simulink model "GFLGFM"  (R2022a)
settings: Solver=FixedStepAuto  StartTime=0.0  StopTime=3  FixedStep=Ts  RelTol=1e-3
values from neighbouring files (symbols this model uses):
  Cf1 = 0.002    [GFLGFM_Para.m]
  Cf2 = 0.2    [GFLGFM_Para.m]
  dt_jump = 2    [GFLGFM_Para.m]    (also in GFLGSP_Para.m)
  dt_sag = 0.01    [GFLGFM_Para.m]    (also in GFLGSP_Para.m)
  ki_pll1 = 0    [GFLGFM_Para.m]    (also in GFLGSP_Para.m)
  kp_pll1 = w_pll1    [GFLGFM_Para.m]    (also in GFLGSP_Para.m)
  L1 = X1    [GFLGFM_Para.m]    (also in GFLGSP_Para.m)
  L2 = X2    [GFLGFM_Para.m]    (also in GFLGSP_Para.m)
  Lc1 = 1e-9    (= 1e-09)    [GFLGFM_Para.m]
  Lc2 = 1e-9    (= 1e-09)    [GFLGFM_Para.m]
  Lf1 = 0.1    [GFLGFM_Para.m]
  Lf2 = 0.1    [GFLGFM_Para.m]
  Lg = Xg    [GFLGFM_Para.m]    (also in GFLGSP_Para.m)
  M = Kgfm/Wbase    [GFLGFM_Para.m]
  phase_jump = -1.2    [GFLGFM_Para.m]    (also in GFLGSP_Para.m)
  Pm = Pref    [GFLGFM_Para.m]
  position = position    [GFLGSP_Para.m]
  R1 = R1    [GFLGFM_Para.m]    (also in GFLGSP_Para.m)
  R2 = R2    [GFLGFM_Para.m]    (also in GFLGSP_Para.m)
  Rg = Rg    [GFLGFM_Para.m]    (also in GFLGSP_Para.m)
  Sbase = 1    [GFLGFM_Para.m]    (also in GFLGSP_Para.m)
  Scale_ki_v = 60    [GFLGFM_Para.m]
  t0 = 2    [GFLGFM_Para.m]    (also in GFLGSP_Para.m = 2.5)
  t0_jump = 10    [GFLGFM_Para.m]    (also in GFLGSP_Para.m)
  t0_sag = 10    [GFLGFM_Para.m]    (also in GFLGSP_Para.m)
  tc1 = t_c    [GFLGFM_Para.m]    (also in GFLGSP_Para.m = t_c-0.01)
  tc2 = t_c2    [GFLGFM_Para.m]    (also in GFLGSP_Para.m = t_c)
  Ts = 1/Fs    (= 1e-05)    [GFLGFM_Para.m]    (also in GFLGSP_Para.m)
  v_sag = 0.1    [GFLGFM_Para.m]    (also in GFLGSP_Para.m)
  Vbase = 1    [GFLGFM_Para.m]    (also in GFLGSP_Para.m)
  w_droop = 15*2*pi    (= 94.2477796077)    [GFLGFM_Para.m]
  w_i_GFL1 = 2500 *2*pi    (= 15707.9632679)    [GFLGFM_Para.m]    (also in GFLGSP_Para.m = 6283.18530718)
  w_i_GFM = 2500*2*pi    (= 15707.9632679)    [GFLGFM_Para.m]
  w_pll1 = k1p    [GFLGFM_Para.m]    (also in GFLGSP_Para.m)
  w_tau1 = 1e3*2*pi    (= 6283.18530718)    [GFLGFM_Para.m]    (also in GFLGSP_Para.m)
  w_v_GFM = 200 *2*pi    (= 1256.63706144)    [GFLGFM_Para.m]
  Wbase = 2*pi*50    (= 314.159265359)    [GFLGFM_Para.m]    (also in GFLGSP_Para.m)
  Zbase = Vbase/Ibase    (= 1)    [GFLGFM_Para.m]    (also in GFLGSP_Para.m)
undefined symbols (not defined in the file or in its folder): DiscIntNeverNeededParam, I1d, I1q, initial
libraries: spsVoltageMeasurementLib x96, spsCurrentMeasurementLib x78, SimplexPS x36, spsThreePhaseSeriesRLCBranchLib x34, spsControlledVoltageSourceLib x30, SimplexPS_2015a x12, spsGroundLib x7, spsSeriesRLCBranchLib x6, spsThreePhaseBreakerLib x4, spsMultimeterLib x2, spsThreePhaseFaultLib x2, spspowerguiLib x1
(part 1 of 6)
settings Model: Creator=admin_user  LastModifiedBy=yz7521
settings SolverCC: AlgebraicLoopSolver=TrustRegion
settings DataIOCC: ReturnWorkspaceOutputs=off
settings DebuggingCC: UnconnectedInputMsg=warning  UnconnectedOutputMsg=warning  UnconnectedLineMsg=warning  SFMachineParentedDataDiag=warning
settings RTWCC: DLArmComputeVersion=19.05

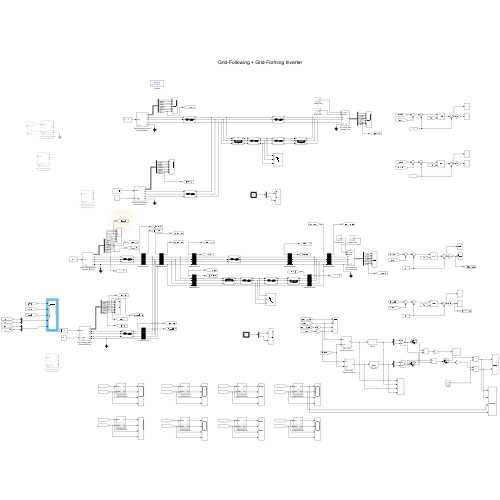
[thumbnail: Simulink's stored preview of the top-level diagram]
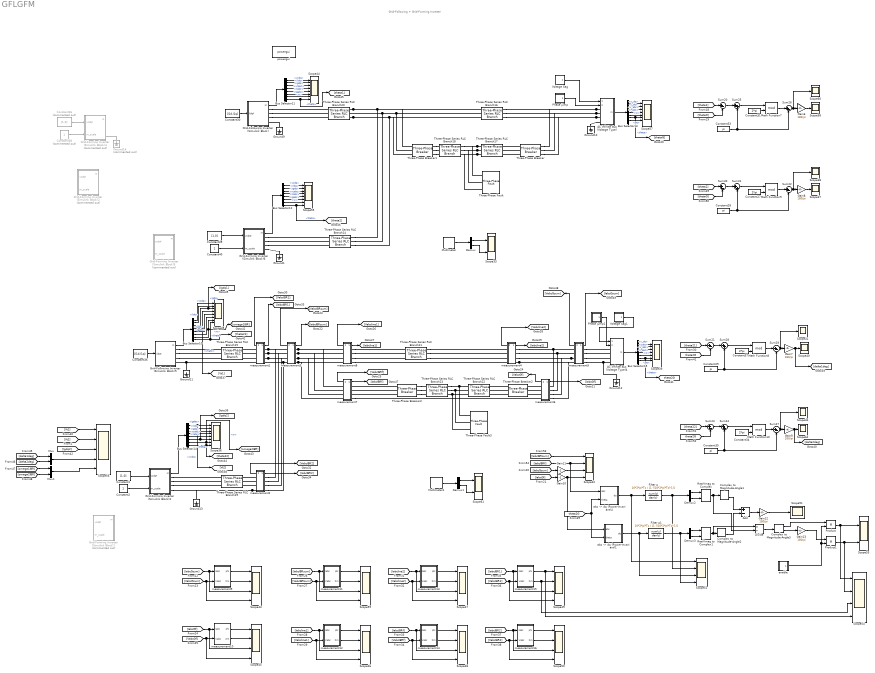
== system GFLGFM ==
  note: Grid-Following + Grid-Forming Inverter
  AC Infinite Bus (Voltage Type) : Subsystem  AncestorBlock=|  mask{Ts=Ts, Sbase=Sbase, Vbase=Vbase, Wbase=Wbase, theta0=0, w=Wbase, R=1e-30}
      | SimplusGT/AC Infinite Bus
      | (Voltage Type)
      mask prompts: Ts "Ts (s), samping period"; Sbase "Sbase (VA), power base"; Vbase "Vbase (V), voltage base"; Wbase "Wbase (rad/s), frequency base"; theta0 "theta0 (rad), initial angle"; w "w (rad/s), frequency"; R "R (Ohm), resistance"
  AC Infinite Bus (Voltage Type)4 : Subsystem  AncestorBlock=|  mask{Ts=Ts, Sbase=Sbase, Vbase=Vbase, Wbase=Wbase, theta0=0, w=Wbase, R=1e-30}
      | SimplusGT/AC Infinite Bus
      | (Voltage Type)
      mask prompts: Ts "Ts (s), samping period"; Sbase "Sbase (VA), power base"; Vbase "Vbase (V), voltage base"; Wbase "Wbase (rad/s), frequency base"; theta0 "theta0 (rad), initial angle"; w "w (rad/s), frequency"; R "R (Ohm), resistance"
  Add : Sum  Inputs=+-
  Bus Selector{10..12,14} (4 alike) : BusSelector  OutputSignals=vcdq,ildq,igdq,vcabc,ilabc,igabc,w,theta
  Bus Selector13 : BusSelector  OutputSignals=v_dq,i_dq,v_abc,i_abc,w,theta,pq
  Bus Selector15 : BusSelector  OutputSignals=v_dq,i_dq,v_abc,i_abc,w,theta,pq
  Complex to Magnitude-Angle1 : ComplexToMagnitudeAngle
  Complex to Magnitude-Angle2 : ComplexToMagnitudeAngle
  Complex to Magnitude-Angle3 : ComplexToMagnitudeAngle
  Constant1 : Constant  Value=[1,0]
  Constant2 : Constant
  Constant26 : Constant  Commented=on  Value=[1,0]
  Constant{27,31,34,37} (4 alike) : Constant  Value=2*pi
  Constant{28..29,33,35} (4 alike) : Constant  Value=pi
  Constant30 : Constant  Value=[I1d,I1q]
  Constant36 : Constant  Value=[I1d,I1q]
  Constant38 : Constant  Commented=on
  Constant39 : Constant  Value=[1,0]
  Constant40 : Constant
  Demux : Demux  Outputs=[3 3]
  Demux1 : Demux  Outputs=[3 3]
  Demux2 : Demux  Outputs=2
  Demux3 : Demux  Outputs=2
  Divide : Product  Inputs=*/
  Filter p : DiscreteTransferFcn  Numerator=10*2*pi*Ts  Denominator=[1 ((10*2*pi*Ts)-1)]  SampleTime=Ts
  Filter p1 : DiscreteTransferFcn  Numerator=10*2*pi*Ts  Denominator=[1 ((10*2*pi*Ts)-1)]  SampleTime=Ts
  Gain10 : Gain  Gain=-1
  Gain11 : Gain  Gain=-1
  Gain{6..9,12..13} (6 alike) : Gain  Gain=180/pi
  Grid-Following Inverter (Simulink Block) : Subsystem  AncestorBlock=|  mask{Ts=Ts, Sbase=Sbase, Vbase=Vbase, Wbase=Wbase, w_i=w_i_GFL1, w_pll=w_pll1, w_tau=w_tau1, Lf=Lf1, Cf=Cf1, Lc=Lc1}
      | SimplusGT/Grid-Following Inverter
      | (Simulink Block)
      mask prompts: Ts "Ts (s), sampling period"; Sbase "Sbase (VA), base power"; Vbase "Vbase (V), base voltage"; Wbase "Wbase (rad/s), base frequency"; w_i "w_i (rad/s), current-loop bandwidth"; w_pll "w_pll (rad/s), PLL bandwidth"; w_tau "w_tau (rad/s), PLL filter bandwidth"; Lf "Lf (pu), LCL filter"; Cf "Cf (pu), LCL filter"; Lc "Lc (pu), LCL filter"
  Grid-Following Inverter (Simulink Block)5 : Subsystem  AncestorBlock=|  mask{Ts=Ts, Sbase=Sbase, Vbase=Vbase, Wbase=Wbase, w_i=w_i_GFL1, w_pll=w_pll1, w_tau=w_tau1, Lf=Lf1, Cf=Cf1, Lc=Lc1}
      | SimplusGT/Grid-Following Inverter
      | (Simulink Block)
      mask prompts: Ts "Ts (s), sampling period"; Sbase "Sbase (VA), base power"; Vbase "Vbase (V), base voltage"; Wbase "Wbase (rad/s), base frequency"; w_i "w_i (rad/s), current-loop bandwidth"; w_pll "w_pll (rad/s), PLL bandwidth"; w_tau "w_tau (rad/s), PLL filter bandwidth"; Lf "Lf (pu), LCL filter"; Cf "Cf (pu), LCL filter"; Lc "Lc (pu), LCL filter"
  Grid-Forming Inverter (Simulink Block)1 : Subsystem  Commented=on  AncestorBlock=|  mask{Ts=Ts, Sbase=Sbase, Vbase=Vbase, Wbase=Wbase, w_i=w_i_GFM, w_v=w_v_GFM, w_droop=w_droop*1, m=M*1, Lf=Lf2, Cf=Cf2, Lc=Lc2, Scale_ki_v=Scale_ki_v}
      | SimplexPS/Grid-Forming Inverter
      | (Simulink Block)
      mask prompts: Ts "Ts (s), sampling period"; Sbase "Sbase (VA), base power"; Vbase "Vbase (V), base voltage"; Wbase "Wbase (rad/s), base frequency"; w_i "w_i (rad/s), current-loop bandwidth"; w_v "w_v (rad/s), voltage-loop bandwidth"; w_droop "w_droop (rad/s), droop bandwidth"; m "m (pu), frequency droop gain"; Lf "Lf (pu), LCL filter"; Cf "Cf (pu), LCL filter"; Lc "Lc (pu), LCL filter"
  Grid-Forming Inverter (Simulink Block)2 : Subsystem  Commented=on  AncestorBlock=|  mask{Ts=Ts, Sbase=Sbase, Vbase=Vbase, Wbase=Wbase, w_i=w_i_GFM, w_v=w_v_GFM, w_droop=w_droop*1, m=M*1, Lf=Lf2, Cf=Cf2, Lc=Lc2, Scale_ki_v=Scale_ki_v}
      | SimplexPS/Grid-Forming Inverter
      | (Simulink Block)
      mask prompts: Ts "Ts (s), sampling period"; Sbase "Sbase (VA), base power"; Vbase "Vbase (V), base voltage"; Wbase "Wbase (rad/s), base frequency"; w_i "w_i (rad/s), current-loop bandwidth"; w_v "w_v (rad/s), voltage-loop bandwidth"; w_droop "w_droop (rad/s), droop bandwidth"; m "m (pu), frequency droop gain"; Lf "Lf (pu), LCL filter"; Cf "Cf (pu), LCL filter"; Lc "Lc (pu), LCL filter"
  Grid-Forming Inverter (Simulink Block)3 : Subsystem  AncestorBlock=|  mask{Ts=Ts, Sbase=Sbase, Vbase=Vbase, Wbase=Wbase, w_i=w_i_GFM, w_v=w_v_GFM, w_droop=w_droop*1, m=M*1, Lf=Lf2, Cf=Cf2, Lc=Lc2, Scale_ki_v=Scale_ki_v}
      | SimplexPS/Grid-Forming Inverter
      | (Simulink Block)
      mask prompts: Ts "Ts (s), sampling period"; Sbase "Sbase (VA), base power"; Vbase "Vbase (V), base voltage"; Wbase "Wbase (rad/s), base frequency"; w_i "w_i (rad/s), current-loop bandwidth"; w_v "w_v (rad/s), voltage-loop bandwidth"; w_droop "w_droop (rad/s), droop bandwidth"; m "m (pu), frequency droop gain"; Lf "Lf (pu), LCL filter"; Cf "Cf (pu), LCL filter"; Lc "Lc (pu), LCL filter"
  Grid-Forming Inverter (Simulink Block)4 : Subsystem  Commented=on  AncestorBlock=|  mask{Ts=Ts, Sbase=Sbase, Vbase=Vbase, Wbase=Wbase, w_i=w_i_GFM, w_v=w_v_GFM, w_droop=w_droop*1, m=M*1, Lf=Lf2, Cf=Cf2, Lc=Lc2, Scale_ki_v=Scale_ki_v}
      | SimplexPS/Grid-Forming Inverter
      | (Simulink Block)
      mask prompts: Ts "Ts (s), sampling period"; Sbase "Sbase (VA), base power"; Vbase "Vbase (V), base voltage"; Wbase "Wbase (rad/s), base frequency"; w_i "w_i (rad/s), current-loop bandwidth"; w_v "w_v (rad/s), voltage-loop bandwidth"; w_droop "w_droop (rad/s), droop bandwidth"; m "m (pu), frequency droop gain"; Lf "Lf (pu), LCL filter"; Cf "Cf (pu), LCL filter"; Lc "Lc (pu), LCL filter"
  Grid-Forming Inverter (Simulink Block)5 : Subsystem  Commented=on  AncestorBlock=|  mask{Ts=Ts, Sbase=Sbase, Vbase=Vbase, Wbase=Wbase, w_i=w_i_GFM, w_v=w_v_GFM, w_droop=w_droop*1, m=M*1, Lf=Lf2, Cf=Cf2, Lc=Lc2, Scale_ki_v=Scale_ki_v}
      | SimplexPS/Grid-Forming Inverter
      | (Simulink Block)
      mask prompts: Ts "Ts (s), sampling period"; Sbase "Sbase (VA), base power"; Vbase "Vbase (V), base voltage"; Wbase "Wbase (rad/s), base frequency"; w_i "w_i (rad/s), current-loop bandwidth"; w_v "w_v (rad/s), voltage-loop bandwidth"; w_droop "w_droop (rad/s), droop bandwidth"; m "m (pu), frequency droop gain"; Lf "Lf (pu), LCL filter"; Cf "Cf (pu), LCL filter"; Lc "Lc (pu), LCL filter"
  Grid-Forming Inverter (Simulink Block)6 : Subsystem  AncestorBlock=|  mask{Ts=Ts, Sbase=Sbase, Vbase=Vbase, Wbase=Wbase, w_i=w_i_GFM, w_v=w_v_GFM, w_droop=w_droop*1, m=M*1, Lf=Lf2, Cf=Cf2, Lc=Lc2, Scale_ki_v=Scale_ki_v}
      | SimplexPS/Grid-Forming Inverter
      | (Simulink Block)
      mask prompts: Ts "Ts (s), sampling period"; Sbase "Sbase (VA), base power"; Vbase "Vbase (V), base voltage"; Wbase "Wbase (rad/s), base frequency"; w_i "w_i (rad/s), current-loop bandwidth"; w_v "w_v (rad/s), voltage-loop bandwidth"; w_droop "w_droop (rad/s), droop bandwidth"; m "m (pu), frequency droop gain"; Lf "Lf (pu), LCL filter"; Cf "Cf (pu), LCL filter"; Lc "Lc (pu), LCL filter"
  Ground{1,9..13} (6 alike) : spsGroundLib/Ground  LConnTagsString=a
  Ground14 : spsGroundLib/Ground  Commented=on  LConnTagsString=a
  Math Function{7..10} (4 alike) : Math  Operator=mod  SignedPower=on
  Multimeter : spsMultimeterLib/Multimeter  L=12  sel=[1 2 3 4 5 6]  yselected={}  Gain=[1 1 1 1 1 1]  OutputType=Complex  PlotAtSimulationStop=off  PhasorSimulation=off
  Multimeter1 : spsMultimeterLib/Multimeter  L=12  sel=[7 8 9 10 11 12]  yselected={}  Gain=[1 1 1 1 1 1]  OutputType=Complex  PlotAtSimulationStop=off  PhasorSimulation=off
  Mux : Mux  Inputs=2
  Mux1 : Mux  Inputs=2
  Phase jump : Subsystem  AncestorBlock=SimplusGT/Single Pulse  mask{t0=t0_jump, dt=dt_jump, Am=phase_jump}
      mask prompts: t0 "t0 (s), starting time"; dt "dt (s), pulse width"; Am "Am, pulse amplitude"
  Phase jump1 : Subsystem  AncestorBlock=SimplusGT/Single Pulse  mask{t0=t0_jump, dt=dt_jump, Am=phase_jump}
      mask prompts: t0 "t0 (s), starting time"; dt "dt (s), pulse width"; Am "Am, pulse amplitude"
  Product : Product
  Product1 : Product
  Real-Imag to Complex : RealImagToComplex
  Real-Imag to Complex1 : RealImagToComplex
  Scope33 : Scope  NumInputPorts=2
  Scope{34,37..38,40..41,51,58,60,62} (9 alike) : Scope
  Scope{35..36,39,44,55,57} (6 alike) : Scope  NumInputPorts=8
  Scope{42..43,45..50,52,54,59} (11 alike) : Scope  NumInputPorts=4
  Scope53 : Scope  NumInputPorts=2
  Scope56 : Scope  NumInputPorts=5
  Scope61 : Scope  NumInputPorts=2
  Sum{20..23,26..27,29..30} (8 alike) : Sum  Inputs=|+-
  Sum{24..25,28,31} (4 alike) : Sum  Inputs=|++
  Three-Phase Series RLC Branch14 : spsThreePhaseSeriesRLCBranchLib/Three-Phase Series RLC Branch  LConnTagsString=A|B|C  RConnTagsString=A|B|C  BranchType=RL  Resistance=R2*Zbase  Inductance=L2*Zbase/Wbase  Capacitance=1/Wbase  Measurements=None
  Three-Phase Series RLC Branch15 : spsThreePhaseSeriesRLCBranchLib/Three-Phase Series RLC Branch  LConnTagsString=A|B|C  RConnTagsString=A|B|C  BranchType=RL  Resistance=R1*Zbase  Inductance=L1*Zbase/Wbase  Capacitance=1/Wbase  Measurements=None
  Three-Phase Series RLC Branch16 : spsThreePhaseSeriesRLCBranchLib/Three-Phase Series RLC Branch  LConnTagsString=A|B|C  RConnTagsString=A|B|C  BranchType=RL  Resistance=Rg*Zbase  Inductance=Lg*Zbase/Wbase  Capacitance=1/Wbase  Measurements=None
  Three-Phase Series RLC Branch17 : spsThreePhaseSeriesRLCBranchLib/Three-Phase Series RLC Branch  LConnTagsString=A|B|C  RConnTagsString=A|B|C  BranchType=RL  Resistance=Rg*Zbase*position  Inductance=Lg*Zbase/Wbase*position  Capacitance=1/Wbase  Measurements=None
  Three-Phase Series RLC Branch18 : spsThreePhaseSeriesRLCBranchLib/Three-Phase Series RLC Branch  LConnTagsString=A|B|C  RConnTagsString=A|B|C  BranchType=RL  Resistance=Rg*Zbase*(1-position)  Inductance=Lg*Zbase/Wbase*(1-position)  Capacitance=1/Wbase  Measurements=None
  Three-Phase Series RLC Branch19 : spsThreePhaseSeriesRLCBranchLib/Three-Phase Series RLC Branch  LConnTagsString=A|B|C  RConnTagsString=A|B|C  BranchType=RL  Resistance=R2*Zbase  Inductance=L2*Zbase/Wbase  Capacitance=1/Wbase  Measurements=None
  Three-Phase Series RLC Branch20 : spsThreePhaseSeriesRLCBranchLib/Three-Phase Series RLC Branch  LConnTagsString=A|B|C  RConnTagsString=A|B|C  BranchType=RL  Resistance=R1*Zbase  Inductance=L1*Zbase/Wbase  Capacitance=1/Wbase  Measurements=None
  Three-Phase Series RLC Branch21 : spsThreePhaseSeriesRLCBranchLib/Three-Phase Series RLC Branch  LConnTagsString=A|B|C  RConnTagsString=A|B|C  BranchType=RL  Resistance=Rg*Zbase  Inductance=Lg*Zbase/Wbase  Capacitance=1/Wbase  Measurements=None
  Three-Phase Series RLC Branch22 : spsThreePhaseSeriesRLCBranchLib/Three-Phase Series RLC Branch  LConnTagsString=A|B|C  RConnTagsString=A|B|C  BranchType=RL  Resistance=Rg*Zbase*position  Inductance=Lg*Zbase/Wbase*position  Capacitance=1/Wbase  Measurements=None
  Three-Phase Series RLC Branch23 : spsThreePhaseSeriesRLCBranchLib/Three-Phase Series RLC Branch  LConnTagsString=A|B|C  RConnTagsString=A|B|C  BranchType=RL  Resistance=Rg*Zbase*(1-position)  Inductance=Lg*Zbase/Wbase*(1-position)  Capacitance=1/Wbase  Measurements=None
  Three-Phase Breaker : spsThreePhaseBreakerLib/Three-Phase Breaker  InitialState=closed  SwitchA=on  SwitchB=on  SwitchC=on  SwitchTimes=[t0+tc1]  External=off  BreakerResistance=0.01e-3  SnubberResistance=1e8  SnubberCapacitance=inf  Measurements=Breaker currents
  Three-Phase Breaker1 : spsThreePhaseBreakerLib/Three-Phase Breaker  InitialState=closed  SwitchA=on  SwitchB=on  SwitchC=on  SwitchTimes=[t0+tc1]  External=off  BreakerResistance=0.01e-3  SnubberResistance=1e8  SnubberCapacitance=inf  Measurements=Breaker currents
  Three-Phase Breaker2 : spsThreePhaseBreakerLib/Three-Phase Breaker  InitialState=closed  SwitchA=on  SwitchB=on  SwitchC=on  SwitchTimes=[t0+tc2]  External=off  BreakerResistance=0.01e-3  SnubberResistance=1e8  SnubberCapacitance=inf  Measurements=Breaker currents
  Three-Phase Breaker3 : spsThreePhaseBreakerLib/Three-Phase Breaker  InitialState=closed  SwitchA=on  SwitchB=on  SwitchC=on  SwitchTimes=t0+tc2  External=off  BreakerResistance=0.01e-3  SnubberResistance=1e10  SnubberCapacitance=inf  Measurements=Breaker currents
  Three-Phase Fault : spsThreePhaseFaultLib/Three-Phase Fault  InitialStates=0  FaultA=on  FaultB=on  FaultC=on  GroundFault=on  SwitchTimes=[t0]  External=off  SwitchStatus=NaN  FaultResistance=Rf  GroundResistance=0.01e-6  SnubberResistance=10e6  SnubberCapacitance=inf  Measurements=None
  Three-Phase Fault3 : spsThreePhaseFaultLib/Three-Phase Fault  InitialStates=0  FaultA=on  FaultB=on  FaultC=on  GroundFault=on  SwitchTimes=[t0]  External=off  SwitchStatus=NaN  FaultResistance=1e-9  GroundResistance=0.01e-6  SnubberResistance=10e6  SnubberCapacitance=inf  Measurements=None
  Voltage Sag : Subsystem  AncestorBlock=SimplusGT/Single Pulse  mask{t0=t0_sag, dt=dt_sag, Am=v_sag}
      mask prompts: t0 "t0 (s), starting time"; dt "dt (s), pulse width"; Am "Am, pulse amplitude"
  Voltage Sag1 : Subsystem  AncestorBlock=SimplusGT/Single Pulse  mask{t0=t0_sag, dt=dt_sag, Am=v_sag}
      mask prompts: t0 "t0 (s), starting time"; dt "dt (s), pulse width"; Am "Am, pulse amplitude"
  "abc -> dq (Power-Invariant)1" : Subsystem  AncestorBlock=|
      | SimplusGT/abc -> dq
      | (Power-Invariant)
  "abc -> dq (Power-Invariant)4" : Subsystem  AncestorBlock=|
      | SimplusGT/abc -> dq
      | (Power-Invariant)
  enable : Subsystem  AncestorBlock=SimplusGT/Single Pulse  mask{t0=0, dt=tc2+t0, Am=1}
      mask prompts: t0 "t0 (s), starting time"; dt "dt (s), pulse width"; Am "Am, pulse amplitude"
  measurement1 : Subsystem
      settings: PortSchema="{\"entries\":[{\"content\":{\"sides\":[{\"content\":{\"connectorIds\":[\"Out2\",\"LConn1\",\"LConn2\",\"LConn3\",\"LConn4\"]},\"type\":\"ConnectorPlacement.EquallySpacedRectSide\",\"uuid\":\"b97639c7-89ad-4c11-8fcc-ddc4f61f4533\"},{\"content\":{\"connectorIds\":[\"Out1\",\"RConn1\",\"RConn2\",\"RConn3\",\"RConn4\"],\"side\":\"RIGHT\"},\"type\":\"ConnectorPlacement.EquallySpacedRectSide\",\"uuid\":\"3b8f0759-83d7-4d3a-a5c5-bdf29e7cbe5b\"},{\"content\":{\"connectorIds\":[],\"side\":\"TOP\"},\"type\":\"ConnectorPlacement.EquallySpacedRectSide\",\"uuid\":\"1e391932-f1e1-4127-bfe0-28b7de5de667\"},{\"content\":{\"connectorIds\":[],\"side\":\"BOTTOM\"},\"type\":\"ConnectorPlacement.EquallySpacedRectSide\",\"uuid\":\"f0c236e9-048a-4270-a45f-ff2fecf0ec8b\"}]},\"type\":\"ConnectorPlacement.EquallySpacedConnector\",\"uuid\":\"002609f8-6c16-431f-ae58-b6d94c927972\"}],\"packageUris\":[\"http://schema.mathworks.com/mf0/Connector/R2020b\"],\"version\":\"1.0\"}"
  measurement10 : Subsystem
  measurement11 : Subsystem
  measurement12 : Subsystem
  measurement13 : Subsystem
  measurement14 : Subsystem
  measurement15 : Subsystem
  measurement16 : Subsystem
  measurement2 : Subsystem
      settings: PortSchema="{\"entries\":[{\"content\":{\"sides\":[{\"content\":{\"connectorIds\":[\"Out2\",\"LConn1\",\"LConn2\",\"LConn3\",\"LConn4\"]},\"type\":\"ConnectorPlacement.EquallySpacedRectSide\",\"uuid\":\"b97639c7-89ad-4c11-8fcc-ddc4f61f4533\"},{\"content\":{\"connectorIds\":[\"Out1\",\"RConn1\",\"RConn2\",\"RConn3\",\"RConn4\"],\"side\":\"RIGHT\"},\"type\":\"ConnectorPlacement.EquallySpacedRectSide\",\"uuid\":\"3b8f0759-83d7-4d3a-a5c5-bdf29e7cbe5b\"},{\"content\":{\"connectorIds\":[],\"side\":\"TOP\"},\"type\":\"ConnectorPlacement.EquallySpacedRectSide\",\"uuid\":\"1e391932-f1e1-4127-bfe0-28b7de5de667\"},{\"content\":{\"connectorIds\":[],\"side\":\"BOTTOM\"},\"type\":\"ConnectorPlacement.EquallySpacedRectSide\",\"uuid\":\"f0c236e9-048a-4270-a45f-ff2fecf0ec8b\"}]},\"type\":\"ConnectorPlacement.EquallySpacedConnector\",\"uuid\":\"002609f8-6c16-431f-ae58-b6d94c927972\"}],\"packageUris\":[\"http://schema.mathworks.com/mf0/Connector/R2020b\"],\"version\":\"1.0\"}"
  measurement3 : Subsystem
      settings: PortSchema="{\"entries\":[{\"content\":{\"sides\":[{\"content\":{\"connectorIds\":[\"Out2\",\"LConn1\",\"LConn2\",\"LConn3\",\"LConn4\"]},\"type\":\"ConnectorPlacement.EquallySpacedRectSide\",\"uuid\":\"b97639c7-89ad-4c11-8fcc-ddc4f61f4533\"},{\"content\":{\"connectorIds\":[\"Out1\",\"RConn1\",\"RConn2\",\"RConn3\",\"RConn4\"],\"side\":\"RIGHT\"},\"type\":\"ConnectorPlacement.EquallySpacedRectSide\",\"uuid\":\"3b8f0759-83d7-4d3a-a5c5-bdf29e7cbe5b\"},{\"content\":{\"connectorIds\":[],\"side\":\"TOP\"},\"type\":\"ConnectorPlacement.EquallySpacedRectSide\",\"uuid\":\"1e391932-f1e1-4127-bfe0-28b7de5de667\"},{\"content\":{\"connectorIds\":[],\"side\":\"BOTTOM\"},\"type\":\"ConnectorPlacement.EquallySpacedRectSide\",\"uuid\":\"f0c236e9-048a-4270-a45f-ff2fecf0ec8b\"}]},\"type\":\"ConnectorPlacement.EquallySpacedConnector\",\"uuid\":\"002609f8-6c16-431f-ae58-b6d94c927972\"}],\"packageUris\":[\"http://schema.mathworks.com/mf0/Connector/R2020b\"],\"version\":\"1.0\"}"
  measurement4 : Subsystem
      settings: PortSchema="{\"entries\":[{\"content\":{\"sides\":[{\"content\":{\"connectorIds\":[\"Out2\",\"LConn1\",\"LConn2\",\"LConn3\",\"LConn4\"]},\"type\":\"ConnectorPlacement.EquallySpacedRectSide\",\"uuid\":\"b97639c7-89ad-4c11-8fcc-ddc4f61f4533\"},{\"content\":{\"connectorIds\":[\"Out1\",\"RConn1\",\"RConn2\",\"RConn3\",\"RConn4\"],\"side\":\"RIGHT\"},\"type\":\"ConnectorPlacement.EquallySpacedRectSide\",\"uuid\":\"3b8f0759-83d7-4d3a-a5c5-bdf29e7cbe5b\"},{\"content\":{\"connectorIds\":[],\"side\":\"TOP\"},\"type\":\"ConnectorPlacement.EquallySpacedRectSide\",\"uuid\":\"1e391932-f1e1-4127-bfe0-28b7de5de667\"},{\"content\":{\"connectorIds\":[],\"side\":\"BOTTOM\"},\"type\":\"ConnectorPlacement.EquallySpacedRectSide\",\"uuid\":\"f0c236e9-048a-4270-a45f-ff2fecf0ec8b\"}]},\"type\":\"ConnectorPlacement.EquallySpacedConnector\",\"uuid\":\"002609f8-6c16-431f-ae58-b6d94c927972\"}],\"packageUris\":[\"http://schema.mathworks.com/mf0/Connector/R2020b\"],\"version\":\"1.0\"}"
  measurement5 : Subsystem
      settings: PortSchema="{\"entries\":[{\"content\":{\"sides\":[{\"content\":{\"connectorIds\":[\"Out2\",\"LConn1\",\"LConn2\",\"LConn3\",\"LConn4\"]},\"type\":\"ConnectorPlacement.EquallySpacedRectSide\",\"uuid\":\"b97639c7-89ad-4c11-8fcc-ddc4f61f4533\"},{\"content\":{\"connectorIds\":[\"Out1\",\"RConn1\",\"RConn2\",\"RConn3\",\"RConn4\"],\"side\":\"RIGHT\"},\"type\":\"ConnectorPlacement.EquallySpacedRectSide\",\"uuid\":\"3b8f0759-83d7-4d3a-a5c5-bdf29e7cbe5b\"},{\"content\":{\"connectorIds\":[],\"side\":\"TOP\"},\"type\":\"ConnectorPlacement.EquallySpacedRectSide\",\"uuid\":\"1e391932-f1e1-4127-bfe0-28b7de5de667\"},{\"content\":{\"connectorIds\":[],\"side\":\"BOTTOM\"},\"type\":\"ConnectorPlacement.EquallySpacedRectSide\",\"uuid\":\"f0c236e9-048a-4270-a45f-ff2fecf0ec8b\"}]},\"type\":\"ConnectorPlacement.EquallySpacedConnector\",\"uuid\":\"002609f8-6c16-431f-ae58-b6d94c927972\"}],\"packageUris\":[\"http://schema.mathworks.com/mf0/Connector/R2020b\"],\"version\":\"1.0\"}"
  measurement6 : Subsystem
      settings: PortSchema="{\"entries\":[{\"content\":{\"sides\":[{\"content\":{\"connectorIds\":[\"Out2\",\"LConn1\",\"LConn2\",\"LConn3\",\"LConn4\"]},\"type\":\"ConnectorPlacement.EquallySpacedRectSide\",\"uuid\":\"b97639c7-89ad-4c11-8fcc-ddc4f61f4533\"},{\"content\":{\"connectorIds\":[\"Out1\",\"RConn1\",\"RConn2\",\"RConn3\",\"RConn4\"],\"side\":\"RIGHT\"},\"type\":\"ConnectorPlacement.EquallySpacedRectSide\",\"uuid\":\"3b8f0759-83d7-4d3a-a5c5-bdf29e7cbe5b\"},{\"content\":{\"connectorIds\":[],\"side\":\"TOP\"},\"type\":\"ConnectorPlacement.EquallySpacedRectSide\",\"uuid\":\"1e391932-f1e1-4127-bfe0-28b7de5de667\"},{\"content\":{\"connectorIds\":[],\"side\":\"BOTTOM\"},\"type\":\"ConnectorPlacement.EquallySpacedRectSide\",\"uuid\":\"f0c236e9-048a-4270-a45f-ff2fecf0ec8b\"}]},\"type\":\"ConnectorPlacement.EquallySpacedConnector\",\"uuid\":\"002609f8-6c16-431f-ae58-b6d94c927972\"}],\"packageUris\":[\"http://schema.mathworks.com/mf0/Connector/R2020b\"],\"version\":\"1.0\"}"
  measurement7 : Subsystem
      settings: PortSchema="{\"entries\":[{\"content\":{\"sides\":[{\"content\":{\"connectorIds\":[\"Out2\",\"LConn1\",\"LConn2\",\"LConn3\",\"LConn4\"]},\"type\":\"ConnectorPlacement.EquallySpacedRectSide\",\"uuid\":\"b97639c7-89ad-4c11-8fcc-ddc4f61f4533\"},{\"content\":{\"connectorIds\":[\"Out1\",\"RConn1\",\"RConn2\",\"RConn3\",\"RConn4\"],\"side\":\"RIGHT\"},\"type\":\"ConnectorPlacement.EquallySpacedRectSide\",\"uuid\":\"3b8f0759-83d7-4d3a-a5c5-bdf29e7cbe5b\"},{\"content\":{\"connectorIds\":[],\"side\":\"TOP\"},\"type\":\"ConnectorPlacement.EquallySpacedRectSide\",\"uuid\":\"1e391932-f1e1-4127-bfe0-28b7de5de667\"},{\"content\":{\"connectorIds\":[],\"side\":\"BOTTOM\"},\"type\":\"ConnectorPlacement.EquallySpacedRectSide\",\"uuid\":\"f0c236e9-048a-4270-a45f-ff2fecf0ec8b\"}]},\"type\":\"ConnectorPlacement.EquallySpacedConnector\",\"uuid\":\"002609f8-6c16-431f-ae58-b6d94c927972\"}],\"packageUris\":[\"http://schema.mathworks.com/mf0/Connector/R2020b\"],\"version\":\"1.0\"}"
  measurement8 : Subsystem
      settings: PortSchema="{\"entries\":[{\"content\":{\"sides\":[{\"content\":{\"connectorIds\":[\"Out2\",\"LConn1\",\"LConn2\",\"LConn3\",\"LConn4\"]},\"type\":\"ConnectorPlacement.EquallySpacedRectSide\",\"uuid\":\"b97639c7-89ad-4c11-8fcc-ddc4f61f4533\"},{\"content\":{\"connectorIds\":[\"Out1\",\"RConn1\",\"RConn2\",\"RConn3\",\"RConn4\"],\"side\":\"RIGHT\"},\"type\":\"ConnectorPlacement.EquallySpacedRectSide\",\"uuid\":\"3b8f0759-83d7-4d3a-a5c5-bdf29e7cbe5b\"},{\"content\":{\"connectorIds\":[],\"side\":\"TOP\"},\"type\":\"ConnectorPlacement.EquallySpacedRectSide\",\"uuid\":\"1e391932-f1e1-4127-bfe0-28b7de5de667\"},{\"content\":{\"connectorIds\":[],\"side\":\"BOTTOM\"},\"type\":\"ConnectorPlacement.EquallySpacedRectSide\",\"uuid\":\"f0c236e9-048a-4270-a45f-ff2fecf0ec8b\"}]},\"type\":\"ConnectorPlacement.EquallySpacedConnector\",\"uuid\":\"002609f8-6c16-431f-ae58-b6d94c927972\"}],\"packageUris\":[\"http://schema.mathworks.com/mf0/Connector/R2020b\"],\"version\":\"1.0\"}"
  measurement9 : Subsystem
  powergui : spspowerguiLib/powergui  Priority=1  SimulationMode=Discrete  SampleTime=Ts  frequency=60  Iterations=50  frequencyindice=0  Pbase=100e6  ErrMax=1e-4  UnitsV=kV  UnitsW=MW  buscounter=0  FunctionMessages=off  echomessages=off  EnableUseOfTLC=off  CurrentSourceSwitches=off  DisableSnubberDevices=off  DisableRonSwitches=off  DisableVfSwitches=off  DisplayEquations=off  AutomaticDiscreteSolvers=off  SolverType=Tustin/Backward Euler (TBE)  Interpol=off  ExternalGateDelay=off  methode=off  Ts=100  x0status=blocks  SPID=on  SwTol=0  HookPort=off  NonlinearTolerance=1e-4  nMaxIteration=100  ContinueOnMaxIteration=off  RestoreLinks=warning  ResistiveCurrentMeasurement=off  Frange=[0:2:500]  Ylog=off  Xlog=on  ShowGrid=off  save=off  variable=ZData  structure=0  ZoomFFT=off  StartTime=0.0  cycles=1  DisplayStyle=1  fundamental=60  FreqAxis=off  MaxFrequency=1000  frequencyindicesteady=1  RmsSteady=1  display=off
  tag scope: theta2G=global
  wires:
  measurement6/1(Iabc) -> [IabcGf]
  measurement7/2(Vabc) -> [VabcIBRf]
  [thetaG] -> Sum20/2
  measurement4/2(Vabc) -> [Vabcline2]
  Real-Imag to Complex1/1 -> Divide/1, Complex to Magnitude-Angle2/1
  [delta1deg] -> Mux/1
  [IabcGf] -> Gain10/1
  Bus Selector15/1 -> Scope39/1  "<v_dq>"
  Constant31/1 -> Math Function7/2
  [Iabcline1] -> Scope46/3, measurement12/1(Iabc)
  Demux2/1 -> Real-Imag to Complex/1
  Bus Selector10/7 -> [omega1IBR], Scope35/7  "<w>"
  Real-Imag to Complex/1 -> Divide/2, Complex to Magnitude-Angle1/1
  [theta22] -> Sum23/1
  Mux1/1 -> Scope56/5
  measurement15/2(Zm) -> Scope54/3, Scope49/2
  Sum21/1 -> Sum28/1
  measurement8/1(Iabc) -> [Iabcline1]
  Sum31/1 -> Math Function9/1
  Complex to Magnitude-Angle1/2 -> Add/1
  Gain13/1 -> Product1/1
  "abc -> dq (Power-Invariant)1"/1(dq) -> Scope52/3, Filter p1/1
  [VabcIBR2] -> Scope50/4, measurement16/2(Vabc)
  [VabcGf] -> Scope45/4, measurement10/2(Vabc)
  Product1/1 -> Scope54/2, Scope53/2
  Grid-Forming Inverter (Simulink Block)3/1(m) -> Bus Selector14/1
  Demux3/2 -> Real-Imag to Complex1/2
  Filter p/1 -> Scope52/2, Demux2/1
  [theta2G] -> "abc -> dq (Power-Invariant)4"/2(theta), "abc -> dq (Power-Invariant)1"/2(theta)
  Demux2/2 -> Real-Imag to Complex/2
  Demux3/1 -> Real-Imag to Complex1/1
  Gain9/1 -> [delta2deg], Scope62/1
  [IabcGsum] -> Scope43/3, measurement9/1(Iabc)
  [VabcIBRsum] -> Scope59/4, measurement11/2(Vabc)
  Bus Selector10/6 -> Scope35/6  "<igabc>"
  Bus Selector11/2 -> Scope44/2  "<ildq>"
  Gain12/1 -> Scope51/1
  [VabcIBR1] -> Scope49/4, measurement15/2(Vabc)
  Constant28/1 -> Sum31/2, Sum22/2
  Bus Selector14/3 -> Scope36/3  "<igdq>"
  measurement16/2(Zm) -> Scope50/2
  measurement15/1(phi) -> Scope54/4, Scope49/1
  Gain10/1 -> "abc -> dq (Power-Invariant)1"/1(abc), Scope42/4
  measurement2/1(Iabc) -> [IabcIBR2]
  measurement16/1(phi) -> Scope50/1
  [VabcIBRf] -> Scope48/4, measurement14/2(Vabc)
  [IabcIBRf] -> "abc -> dq (Power-Invariant)4"/1(abc), Scope42/2
  [IabcIBR1] -> Scope49/3, measurement15/1(Iabc)
  measurement14/1(phi) -> Scope48/1
  measurement10/1(phi) -> Scope45/1
  Constant34/1 -> Math Function10/2
  measurement14/2(Zm) -> Scope48/2
  Bus Selector14/2 -> Scope36/2  "<ildq>"
  [IabcIBRsum] -> Scope59/3, measurement11/1(Iabc)
  [Vabcline2] -> Scope47/4, measurement13/2(Vabc)
  Add/1 -> Gain12/1
  measurement3/2(Vabc) -> [VabcIBRsum]
  Complex to Magnitude-Angle2/2 -> Add/2
  measurement11/1(phi) -> Scope59/1
  [omega2IBR] -> Mux1/2
  [IabcGf] -> Scope45/3, measurement10/1(Iabc)
  [Iabcline2] -> Scope47/3, measurement13/1(Iabc)
  measurement12/2(Zm) -> Scope46/2
  Sum23/1 -> Sum24/1
  measurement9/2(Zm) -> Scope43/2
  measurement6/2(Vabc) -> [VabcGf]
  measurement2/2(Vabc) -> [VabcIBR2]
  Bus Selector10/3 -> [Igdq1], Scope35/3  "<igdq>"
  Voltage Sag/1(Out) -> AC Infinite Bus (Voltage Type)/1(v_mag)
  [VabcGsum] -> Scope43/4, measurement9/2(Vabc)
  Gain7/1 -> [delta1deg], Scope40/1
  measurement8/2(Vabc) -> [Vabcline1]
  Demux/2 -> Scope33/2
  measurement5/1(Iabc) -> [IabcGsum]
  [delta2deg] -> Mux/2
  Product/1 -> Scope54/1, Scope53/1
  Voltage Sag1/1(Out) -> AC Infinite Bus (Voltage Type)4/1(v_mag)
  Gain11/1 -> Scope42/3
  Bus Selector13/3 -> Scope57/3  "<v_abc>"
  measurement7/1(Iabc) -> [IabcIBRf]
  [omega1IBR] -> Mux1/1
  [Vt1] -> Scope56/1
  measurement3/1(Iabc) -> [IabcIBRsum]
  [IabcGsum] -> Gain11/1
  Sum28/1 -> Math Function8/1
  Bus Selector15/2 -> Scope39/2  "<i_dq>"
  Bus Selector13/2 -> Scope57/2  "<i_dq>"
  Bus Selector14/1 -> [Vt2], Scope36/1  "<vcdq>"
  Bus Selector15/7 -> Scope39/7  "<pq>"
  Bus Selector10/4 -> [Vt1], Scope35/4  "<vcabc>"
  Phase jump1/1(Out) -> AC Infinite Bus (Voltage Type)4/2(Phase)
  Bus Selector15/5 -> Scope39/5  "<w>"
  Bus Selector10/8 -> [theta21], Scope35/8  "<theta>"
  Math Function8/1 -> Sum29/1
  Constant36/1 -> Grid-Following Inverter (Simulink Block)5/1(ildq*)
  Bus Selector10/1 -> Scope35/1  "<vcdq>"
  Bus Selector15/4 -> Scope39/4  "<i_abc>"
  [theta2G] -> Sum21/2
  Constant37/1 -> Math Function8/2
  Constant29/1 -> Sum28/2, Sum29/2
  AC Infinite Bus (Voltage Type)4/1(m) -> Bus Selector15/1
  Bus Selector14/5 -> Scope36/5  "<ilabc>"
  Phase jump/1(Out) -> AC Infinite Bus (Voltage Type)/2(Phase)
  Bus Selector15/3 -> Scope39/3  "<v_abc>"
  Sum27/1 -> Scope34/1, Gain9/1
  Bus Selector11/8 -> [theta1], Scope44/8  "<theta>"
  [theta21] -> Sum21/1
  Bus Selector10/5 -> Scope35/5  "<ilabc>"
  measurement1/1(Iabc) -> [IabcIBR1]
  Bus Selector13/4 -> Scope57/4  "<i_abc>"
  Multimeter1/1 -> Demux1/1
  measurement10/2(Zm) -> Scope45/2
  Bus Selector14/6 -> [Igdq2], Scope36/6  "<igabc>"
  Bus Selector14/8 -> [theta22], Scope36/8  "<theta>"
  Bus Selector10/2 -> Scope35/2  "<ildq>"
  measurement11/2(Zm) -> Scope59/2
  enable/1(Out) -> Product1/2, Product/2
  Bus Selector13/1 -> Scope57/1  "<v_dq>"
  Constant35/1 -> Sum24/2, Sum27/2
  Filter p1/1 -> Scope52/4, Demux3/1
  Demux/1 -> Scope33/1
  [IabcIBR2] -> Scope50/3, measurement16/1(Iabc)
  Multimeter/1 -> Demux/1
  Bus Selector13/6 -> [thetaG], Scope57/6  "<theta>"
  [thetaG] -> Sum30/2
  Math Function9/1 -> Sum22/1
  Constant27/1 -> Math Function9/2
  Sum24/1 -> Math Function10/1
  Sum30/1 -> Sum31/1
  Complex to Magnitude-Angle3/2 -> Gain13/1
  Sum20/1 -> Sum25/1
  [IabcIBRsum] -> Scope42/1
  Sum26/1 -> Scope60/1, Gain6/1
  [IabcIBRf] -> Scope48/3, measurement14/1(Iabc)
  Grid-Following Inverter (Simulink Block)/1(m) -> Bus Selector11/1
  Sum25/1 -> Math Function7/1
  Math Function7/1 -> Sum26/1
  measurement4/1(Iabc) -> [Iabcline2]
  Bus Selector11/6 -> Scope44/6  "<igabc>"
  Math Function10/1 -> Sum27/1
  Bus Selector11/3 -> Scope44/3  "<igdq>"
  Sum22/1 -> Scope38/1, Gain8/1
  Bus Selector13/7 -> Scope57/7  "<pq>"
  Bus Selector11/7 -> Scope44/7  "<w>"
  Bus Selector11/5 -> Scope44/5  "<ilabc>"
  [theta1] -> Sum20/1
  AC Infinite Bus (Voltage Type)/1(m) -> Bus Selector13/1
  Divide/1 -> Complex to Magnitude-Angle3/1
  Bus Selector11/4 -> Scope44/4  "<vcabc>"
  Constant33/1 -> Sum25/2, Sum26/2
  Bus Selector11/1 -> Scope44/1  "<vcdq>"
  Gain8/1 -> Scope37/1
  "abc -> dq (Power-Invariant)4"/1(dq) -> Scope52/1, Filter p/1
  Demux1/1 -> Scope61/1
  [theta2G] -> Sum23/2
  Bus Selector13/5 -> Scope57/5  "<w>"
  Sum29/1 -> Scope41/1, Gain7/1
  Complex to Magnitude-Angle3/1 -> Product/1
  Gain6/1 -> Scope58/1
  [Vabcline1] -> Scope46/4, measurement12/2(Vabc)
  measurement9/1(phi) -> Scope43/1
  Bus Selector15/6 -> [theta2G], Scope39/6  "<theta>"
  Grid-Following Inverter (Simulink Block)5/1(m) -> Bus Selector10/1
  Constant30/1 -> Grid-Following Inverter (Simulink Block)/1(ildq*)
  measurement12/1(phi) -> Scope46/1
  measurement5/2(Vabc) -> [VabcGsum]
  measurement1/2(Vabc) -> [VabcIBR1]
  measurement13/2(Zm) -> Scope47/2
  [theta2] -> Sum30/1
  Bus Selector14/7 -> [omega2IBR], Scope36/7  "<w>"
  Mux/1 -> Scope56/4
  Bus Selector14/4 -> Scope36/4  "<vcabc>"
  measurement13/1(phi) -> Scope47/1
  Demux1/2 -> Scope61/2
  Constant38/1 -> Grid-Forming Inverter (Simulink Block)4/2(m_scale)
  Constant26/1 -> Grid-Forming Inverter (Simulink Block)4/1(vcdq*)
  Bus Selector12/2 -> Scope55/2  "<ildq>"
  Bus Selector12/5 -> Scope55/5  "<ilabc>"
  Bus Selector12/1 -> Scope55/1  "<vcdq>"
  Bus Selector12/4 -> Scope55/4  "<vcabc>"
  Bus Selector12/8 -> [theta2], Scope55/8  "<theta>"
  Grid-Forming Inverter (Simulink Block)6/1(m) -> Bus Selector12/1
  Bus Selector12/3 -> Scope55/3  "<igdq>"
  Bus Selector12/6 -> Scope55/6  "<igabc>"
  Bus Selector12/7 -> Scope55/7  "<w>"
  Constant39/1 -> Grid-Forming Inverter (Simulink Block)6/1(vcdq*)
  Constant40/1 -> Grid-Forming Inverter (Simulink Block)6/2(m_scale)
  Constant2/1 -> Grid-Forming Inverter (Simulink Block)3/2(m_scale)
  Constant1/1 -> Grid-Forming Inverter (Simulink Block)3/1(vcdq*)
  [Vt2] -> Scope56/2
  [Igdq2] -> Scope56/3
  connections:
  Three-Phase Series RLC Branch20/LConn1 -- Three-Phase Series RLC Branch14/LConn1 -- Three-Phase Breaker1/LConn1 -- Three-Phase Series RLC Branch16/RConn1
  measurement3/RConn3 -- measurement8/LConn3 -- measurement7/LConn3
  Three-Phase Series RLC Branch16/RConn2 -- Three-Phase Series RLC Branch14/LConn2 -- Three-Phase Series RLC Branch20/LConn2 -- Three-Phase Breaker1/LConn2
  Three-Phase Series RLC Branch17/RConn3 -- Three-Phase Series RLC Branch18/LConn3 -- Three-Phase Fault/LConn3
  Three-Phase Fault3/LConn3 -- Three-Phase Series RLC Branch22/RConn3 -- Three-Phase Series RLC Branch23/LConn3
  measurement6/RConn1 -- measurement4/RConn1 -- measurement5/LConn1
  AC Infinite Bus (Voltage Type)/LConn2 -- Three-Phase Series RLC Branch16/LConn2 -- Three-Phase Breaker/RConn2
  measurement1/RConn2 -- measurement3/LConn2 -- measurement2/RConn2
  measurement3/RConn2 -- measurement8/LConn2 -- measurement7/LConn2
  Three-Phase Fault3/LConn2 -- Three-Phase Series RLC Branch22/RConn2 -- Three-Phase Series RLC Branch23/LConn2
  measurement4/RConn4 -- measurement5/LConn4 -- measurement6/RConn4
  measurement6/RConn2 -- measurement4/RConn2 -- measurement5/LConn2
  Three-Phase Fault3/LConn1 -- Three-Phase Series RLC Branch22/RConn1 -- Three-Phase Series RLC Branch23/LConn1
  measurement3/RConn4 -- measurement8/LConn4 -- measurement7/LConn4
  measurement3/RConn1 -- measurement8/LConn1 -- measurement7/LConn1
  AC Infinite Bus (Voltage Type)/LConn1 -- Three-Phase Series RLC Branch16/LConn1 -- Three-Phase Breaker/RConn1
  Three-Phase Series RLC Branch17/RConn2 -- Three-Phase Series RLC Branch18/LConn2 -- Three-Phase Fault/LConn2
  measurement5/LConn3 -- measurement4/RConn3 -- measurement6/RConn3
  measurement1/RConn3 -- measurement3/LConn3 -- measurement2/RConn3
  measurement2/RConn4 -- measurement3/LConn4 -- measurement1/RConn4
  AC Infinite Bus (Voltage Type)/LConn3 -- Three-Phase Series RLC Branch16/LConn3 -- Three-Phase Breaker/RConn3
  Three-Phase Series RLC Branch17/RConn1 -- Three-Phase Series RLC Branch18/LConn1 -- Three-Phase Fault/LConn1
  Three-Phase Series RLC Branch20/LConn3 -- Three-Phase Series RLC Branch14/LConn3 -- Three-Phase Breaker1/LConn3 -- Three-Phase Series RLC Branch16/RConn3
  measurement1/RConn1 -- measurement3/LConn1 -- measurement2/RConn1
  Grid-Following Inverter (Simulink Block)5/RConn1 -- Three-Phase Series RLC Branch15/RConn1
  measurement8/RConn3 -- Three-Phase Series RLC Branch21/RConn3
  Three-Phase Breaker3/LConn2 -- Three-Phase Series RLC Branch23/RConn2
  measurement2/LConn4 -- Grid-Forming Inverter (Simulink Block)3/RConn4 -- Ground13/LConn1
  Three-Phase Series RLC Branch21/LConn1 -- measurement4/LConn1
  Grid-Forming Inverter (Simulink Block)3/RConn1 -- Three-Phase Series RLC Branch19/RConn1
  measurement2/LConn2 -- Three-Phase Series RLC Branch19/LConn2
  measurement2/LConn3 -- Three-Phase Series RLC Branch19/LConn3
  Three-Phase Breaker1/RConn1 -- Three-Phase Series RLC Branch18/RConn1
  measurement6/LConn1 -- Three-Phase Breaker2/RConn1
  Three-Phase Breaker3/LConn3 -- Three-Phase Series RLC Branch23/RConn1
  Grid-Following Inverter (Simulink Block)5/RConn3 -- Three-Phase Series RLC Branch15/RConn3
  measurement5/RConn2 -- AC Infinite Bus (Voltage Type)4/LConn2
  measurement1/LConn1 -- Three-Phase Series RLC Branch15/LConn1
  measurement1/LConn3 -- Three-Phase Series RLC Branch15/LConn3
  Three-Phase Series RLC Branch21/LConn2 -- measurement4/LConn2
  measurement8/RConn1 -- Three-Phase Series RLC Branch21/RConn1
  Grid-Forming Inverter (Simulink Block)6/RConn1 -- Three-Phase Series RLC Branch14/RConn1
  Three-Phase Breaker1/RConn2 -- Three-Phase Series RLC Branch18/RConn2
  Three-Phase Breaker1/RConn3 -- Three-Phase Series RLC Branch18/RConn3
  Three-Phase Breaker/LConn3 -- Three-Phase Series RLC Branch17/LConn3
  Three-Phase Breaker3/RConn3 -- measurement7/RConn1
  measurement5/RConn3 -- AC Infinite Bus (Voltage Type)4/LConn3
  measurement6/LConn2 -- Three-Phase Breaker2/RConn2
  measurement1/LConn2 -- Three-Phase Series RLC Branch15/LConn2
  Grid-Forming Inverter (Simulink Block)3/RConn2 -- Three-Phase Series RLC Branch19/RConn2
  Three-Phase Series RLC Branch21/LConn3 -- measurement4/LConn3
  Grid-Following Inverter (Simulink Block)5/RConn2 -- Three-Phase Series RLC Branch15/RConn2
  Three-Phase Breaker2/LConn2 -- Three-Phase Series RLC Branch22/LConn2
  Three-Phase Breaker3/LConn1 -- Three-Phase Series RLC Branch23/RConn3
  Three-Phase Breaker3/RConn2 -- measurement7/RConn2
  Three-Phase Breaker2/LConn1 -- Three-Phase Series RLC Branch22/LConn1
  Three-Phase Breaker/LConn2 -- Three-Phase Series RLC Branch17/LConn2
  Three-Phase Breaker/LConn1 -- Three-Phase Series RLC Branch17/LConn1
  Grid-Forming Inverter (Simulink Block)6/RConn3 -- Three-Phase Series RLC Branch14/RConn3
  Grid-Following Inverter (Simulink Block)/RConn3 -- Three-Phase Series RLC Branch20/RConn3
  Grid-Forming Inverter (Simulink Block)6/RConn2 -- Three-Phase Series RLC Branch14/RConn2
  Three-Phase Breaker2/LConn3 -- Three-Phase Series RLC Branch22/LConn3
  measurement2/LConn1 -- Three-Phase Series RLC Branch19/LConn1
  Grid-Following Inverter (Simulink Block)/RConn2 -- Three-Phase Series RLC Branch20/RConn2
  measurement5/RConn4 -- Ground12/LConn1 -- AC Infinite Bus (Voltage Type)4/LConn4
  measurement8/RConn2 -- Three-Phase Series RLC Branch21/RConn2
  measurement6/LConn3 -- Three-Phase Breaker2/RConn3
  measurement5/RConn1 -- AC Infinite Bus (Voltage Type)4/LConn1
  Grid-Following Inverter (Simulink Block)/RConn1 -- Three-Phase Series RLC Branch20/RConn1
  measurement8/RConn4 -- measurement4/LConn4
  Three-Phase Breaker3/RConn1 -- measurement7/RConn3
  measurement1/LConn4 -- Ground11/LConn1 -- Grid-Following Inverter (Simulink Block)5/RConn4
  Grid-Forming Inverter (Simulink Block)3/RConn3 -- Three-Phase Series RLC Branch19/RConn3
  measurement7/RConn4 -- measurement6/LConn4
  Ground9/LConn1 -- Grid-Following Inverter (Simulink Block)/RConn4
  AC Infinite Bus (Voltage Type)/LConn4 -- Ground10/LConn1
  Ground14/LConn1 -- Grid-Forming Inverter (Simulink Block)4/RConn4
  Grid-Forming Inverter (Simulink Block)6/RConn4 -- Ground1/LConn1

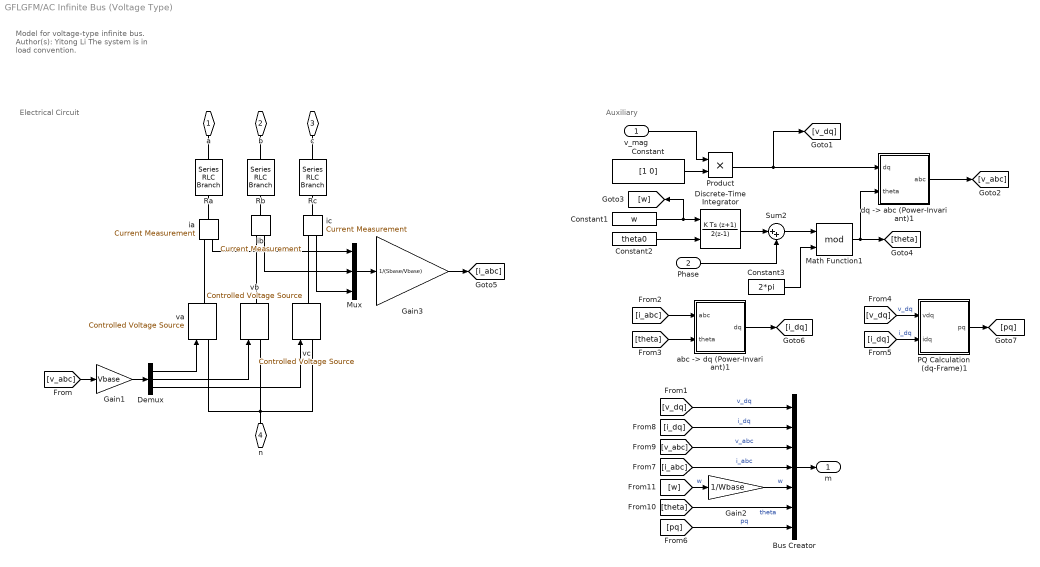
== system GFLGFM/AC Infinite Bus (Voltage Type) ==
  note: Auxiliary
  note: Electrical Circuit
  note: Model for voltage-type infinite bus.
      |
      | Author(s): Yitong Li
      |
      | The system is in load convention.
  v_mag : Inport
  Phase : Inport  Port=2
  Bus Creator : BusCreator  Inputs=7
  Constant : Constant  Value=[1 0]
  Constant1 : Constant  Value=w
  Constant2 : Constant  Value=theta0
  Constant3 : Constant  Value=2*pi
  Demux : Demux  Outputs=3
  Discrete-Time Integrator : DiscreteIntegrator  IntegratorMethod=Integration: Trapezoidal  InitialConditionSource=external  SampleTime=-1  ICPrevOutput=DiscIntNeverNeededParam  ICPrevScaledInput=DiscIntNeverNeededParam
  Gain1 : Gain  Gain=Vbase
  Gain2 : Gain  Gain=1/Wbase
  Gain3 : Gain  Gain=1/(Sbase/Vbase)
  Math Function1 : Math  Operator=mod  SignedPower=on
  Mux : Mux  Inputs=3
  PQ Calculation (dq-Frame)1 : Subsystem  AncestorBlock=|
      | SimplusGT/PQ Calculation
      | (dq-Frame)
  Product : Product
  Ra : spsSeriesRLCBranchLib/Series RLC Branch  LConnTagsString=__new0  RConnTagsString=__new0  BranchType=R  Resistance=R  Inductance=1e-3  SetiL0=off  InitialCurrent=0  Capacitance=1e-6  Setx0=off  InitialVoltage=0  Measurements=None
  Rb : spsSeriesRLCBranchLib/Series RLC Branch  LConnTagsString=__new0  RConnTagsString=__new0  BranchType=R  Resistance=R  Inductance=1e-3  SetiL0=off  InitialCurrent=0  Capacitance=1e-6  Setx0=off  InitialVoltage=0  Measurements=None
  Rc : spsSeriesRLCBranchLib/Series RLC Branch  LConnTagsString=__new0  RConnTagsString=__new0  BranchType=R  Resistance=R  Inductance=1e-3  SetiL0=off  InitialCurrent=0  Capacitance=1e-6  Setx0=off  InitialVoltage=0  Measurements=None
  Sum2 : Sum  Inputs=|++
  "abc -> dq (Power-Invariant)1" : Subsystem  AncestorBlock=|
      | SimplusGT/abc -> dq
      | (Power-Invariant)
  "dq -> abc (Power-Invariant)1" : Subsystem  AncestorBlock=|
      | SimplusGT/dq -> abc
      | (Power-Invariant)
  ia : spsCurrentMeasurementLib/Current Measurement  PhasorSimulation=off  OutputType=Complex  PSBequivalent=0
  ib : spsCurrentMeasurementLib/Current Measurement  PhasorSimulation=off  OutputType=Complex  PSBequivalent=0
  ic : spsCurrentMeasurementLib/Current Measurement  PhasorSimulation=off  OutputType=Complex  PSBequivalent=0
  va : spsControlledVoltageSourceLib/Controlled Voltage Source  Initialize=on  Source_Type=AC  Amplitude=0  Phase=0  Frequency=0  Measurements=None
  vb : spsControlledVoltageSourceLib/Controlled Voltage Source  Initialize=on  Source_Type=AC  Amplitude=0  Phase=0  Frequency=0  Measurements=None
  vc : spsControlledVoltageSourceLib/Controlled Voltage Source  Initialize=on  Source_Type=AC  Amplitude=0  Phase=0  Frequency=0  Measurements=None
  a : PMIOPort  Side=Left
  b : PMIOPort  Port=2  Side=Left
  c : PMIOPort  Port=3  Side=Left
  n : PMIOPort  Port=4  Side=Left
  m : Outport
  wires:
  [pq] -> Bus Creator/7  "pq"
  PQ Calculation (dq-Frame)1/1(pq) -> [pq]
  [i_dq] -> PQ Calculation (dq-Frame)1/2(idq)  "i_dq"
  [v_dq] -> PQ Calculation (dq-Frame)1/1(vdq)  "v_dq"
  Gain3/1 -> [i_abc]
  Mux/1 -> Gain3/1
  Gain1/1 -> Demux/1
  "abc -> dq (Power-Invariant)1"/1(dq) -> [i_dq]
  [theta] -> "abc -> dq (Power-Invariant)1"/2(theta)
  [i_abc] -> "abc -> dq (Power-Invariant)1"/1(abc)
  ic/1 -> Mux/3
  ib/1 -> Mux/2
  ia/1 -> Mux/1
  [theta] -> Bus Creator/6  "theta"
  Bus Creator/1 -> m/1
  [i_dq] -> Bus Creator/2  "i_dq"
  Gain2/1 -> Bus Creator/5  "w"
  [v_abc] -> Bus Creator/3  "v_abc"
  [w] -> Gain2/1  "w"
  [i_abc] -> Bus Creator/4  "i_abc"
  [v_dq] -> Bus Creator/1  "v_dq"
  Constant3/1 -> Math Function1/2
  "dq -> abc (Power-Invariant)1"/1(abc) -> [v_abc]
  Constant1/1 -> [w], Discrete-Time Integrator/1
  Constant2/1 -> Discrete-Time Integrator/2
  Math Function1/1 -> [theta], "dq -> abc (Power-Invariant)1"/2(theta)
  Demux/3 -> vc/1
  Demux/2 -> vb/1
  Demux/1 -> va/1
  [v_abc] -> Gain1/1
  Constant/1 -> Product/2
  v_mag/1 -> Product/1
  Product/1 -> [v_dq], "dq -> abc (Power-Invariant)1"/1(dq)
  Discrete-Time Integrator/1 -> Sum2/1
  Sum2/1 -> Math Function1/1
  Phase/1 -> Sum2/2
  connections:
  Rc/LConn1 -- c/RConn1
  Rc/RConn1 -- ic/LConn1
  Rb/LConn1 -- b/RConn1
  ib/LConn1 -- Rb/RConn1
  Ra/LConn1 -- a/RConn1
  Ra/RConn1 -- ia/LConn1
  ic/RConn1 -- vc/RConn1
  ib/RConn1 -- vb/RConn1
  ia/RConn1 -- va/RConn1
  vb/LConn1 -- va/LConn1 -- n/RConn1 -- vc/LConn1

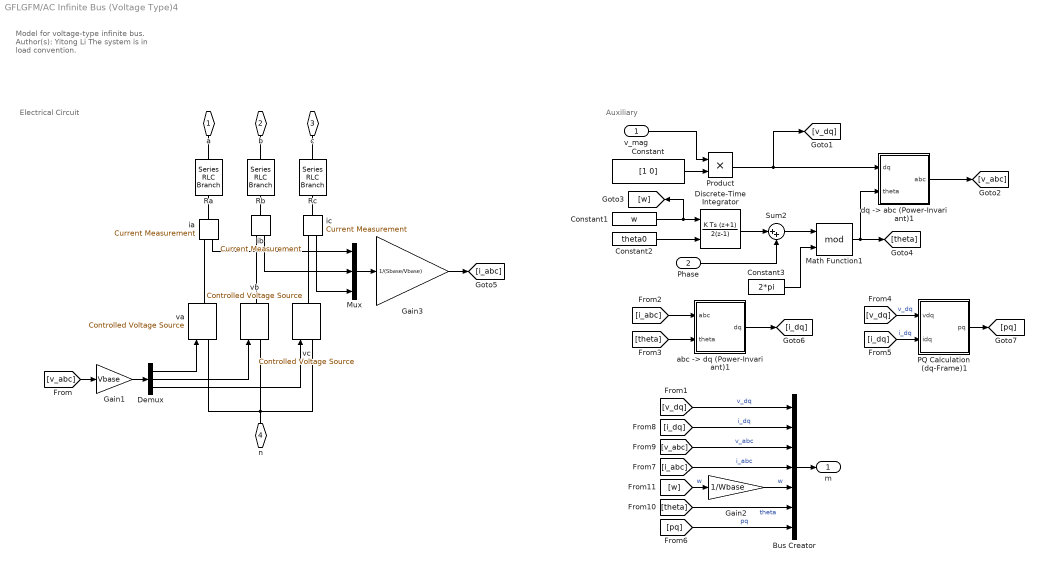
== system GFLGFM/AC Infinite Bus (Voltage Type)4 ==
  note: Auxiliary
  note: Electrical Circuit
  note: Model for voltage-type infinite bus.
      |
      | Author(s): Yitong Li
      |
      | The system is in load convention.
  v_mag : Inport
  Phase : Inport  Port=2
  Bus Creator : BusCreator  Inputs=7
  Constant : Constant  Value=[1 0]
  Constant1 : Constant  Value=w
  Constant2 : Constant  Value=theta0
  Constant3 : Constant  Value=2*pi
  Demux : Demux  Outputs=3
  Discrete-Time Integrator : DiscreteIntegrator  IntegratorMethod=Integration: Trapezoidal  InitialConditionSource=external  SampleTime=-1  ICPrevOutput=DiscIntNeverNeededParam  ICPrevScaledInput=DiscIntNeverNeededParam
  Gain1 : Gain  Gain=Vbase
  Gain2 : Gain  Gain=1/Wbase
  Gain3 : Gain  Gain=1/(Sbase/Vbase)
  Math Function1 : Math  Operator=mod  SignedPower=on
  Mux : Mux  Inputs=3
  PQ Calculation (dq-Frame)1 : Subsystem  AncestorBlock=|
      | SimplusGT/PQ Calculation
      | (dq-Frame)
  Product : Product
  Ra : spsSeriesRLCBranchLib/Series RLC Branch  LConnTagsString=__new0  RConnTagsString=__new0  BranchType=R  Resistance=R  Inductance=1e-3  SetiL0=off  InitialCurrent=0  Capacitance=1e-6  Setx0=off  InitialVoltage=0  Measurements=None
  Rb : spsSeriesRLCBranchLib/Series RLC Branch  LConnTagsString=__new0  RConnTagsString=__new0  BranchType=R  Resistance=R  Inductance=1e-3  SetiL0=off  InitialCurrent=0  Capacitance=1e-6  Setx0=off  InitialVoltage=0  Measurements=None
  Rc : spsSeriesRLCBranchLib/Series RLC Branch  LConnTagsString=__new0  RConnTagsString=__new0  BranchType=R  Resistance=R  Inductance=1e-3  SetiL0=off  InitialCurrent=0  Capacitance=1e-6  Setx0=off  InitialVoltage=0  Measurements=None
  Sum2 : Sum  Inputs=|++
  "abc -> dq (Power-Invariant)1" : Subsystem  AncestorBlock=|
      | SimplusGT/abc -> dq
      | (Power-Invariant)
  "dq -> abc (Power-Invariant)1" : Subsystem  AncestorBlock=|
      | SimplusGT/dq -> abc
      | (Power-Invariant)
  ia : spsCurrentMeasurementLib/Current Measurement  PhasorSimulation=off  OutputType=Complex  PSBequivalent=0
  ib : spsCurrentMeasurementLib/Current Measurement  PhasorSimulation=off  OutputType=Complex  PSBequivalent=0
  ic : spsCurrentMeasurementLib/Current Measurement  PhasorSimulation=off  OutputType=Complex  PSBequivalent=0
  va : spsControlledVoltageSourceLib/Controlled Voltage Source  Initialize=on  Source_Type=AC  Amplitude=0  Phase=0  Frequency=0  Measurements=None
  vb : spsControlledVoltageSourceLib/Controlled Voltage Source  Initialize=on  Source_Type=AC  Amplitude=0  Phase=0  Frequency=0  Measurements=None
  vc : spsControlledVoltageSourceLib/Controlled Voltage Source  Initialize=on  Source_Type=AC  Amplitude=0  Phase=0  Frequency=0  Measurements=None
  a : PMIOPort  Side=Left
  b : PMIOPort  Port=2  Side=Left
  c : PMIOPort  Port=3  Side=Left
  n : PMIOPort  Port=4  Side=Left
  m : Outport
  wires:
  [pq] -> Bus Creator/7  "pq"
  PQ Calculation (dq-Frame)1/1(pq) -> [pq]
  [i_dq] -> PQ Calculation (dq-Frame)1/2(idq)  "i_dq"
  [v_dq] -> PQ Calculation (dq-Frame)1/1(vdq)  "v_dq"
  Gain3/1 -> [i_abc]
  Mux/1 -> Gain3/1
  Gain1/1 -> Demux/1
  "abc -> dq (Power-Invariant)1"/1(dq) -> [i_dq]
  [theta] -> "abc -> dq (Power-Invariant)1"/2(theta)
  [i_abc] -> "abc -> dq (Power-Invariant)1"/1(abc)
  ic/1 -> Mux/3
  ib/1 -> Mux/2
  ia/1 -> Mux/1
  [theta] -> Bus Creator/6  "theta"
  Bus Creator/1 -> m/1
  [i_dq] -> Bus Creator/2  "i_dq"
  Gain2/1 -> Bus Creator/5  "w"
  [v_abc] -> Bus Creator/3  "v_abc"
  [w] -> Gain2/1  "w"
  [i_abc] -> Bus Creator/4  "i_abc"
  [v_dq] -> Bus Creator/1  "v_dq"
  Constant3/1 -> Math Function1/2
  "dq -> abc (Power-Invariant)1"/1(abc) -> [v_abc]
  Constant1/1 -> [w], Discrete-Time Integrator/1
  Constant2/1 -> Discrete-Time Integrator/2
  Math Function1/1 -> [theta], "dq -> abc (Power-Invariant)1"/2(theta)
  Demux/3 -> vc/1
  Demux/2 -> vb/1
  Demux/1 -> va/1
  [v_abc] -> Gain1/1
  Constant/1 -> Product/2
  v_mag/1 -> Product/1
  Product/1 -> [v_dq], "dq -> abc (Power-Invariant)1"/1(dq)
  Discrete-Time Integrator/1 -> Sum2/1
  Sum2/1 -> Math Function1/1
  Phase/1 -> Sum2/2
  connections:
  Rc/LConn1 -- c/RConn1
  Rc/RConn1 -- ic/LConn1
  Rb/LConn1 -- b/RConn1
  ib/LConn1 -- Rb/RConn1
  Ra/LConn1 -- a/RConn1
  Ra/RConn1 -- ia/LConn1
  ic/RConn1 -- vc/RConn1
  ib/RConn1 -- vb/RConn1
  ia/RConn1 -- va/RConn1
  vb/LConn1 -- va/LConn1 -- n/RConn1 -- vc/LConn1
